simulink model "LaneFollowingNMPCWarda"  (R2021b)
settings: Solver=VariableStepAuto  StartTime=0.0  StopTime=Duration  FixedStep=0.1  RelTol=1e-3
PreLoadFcn:
  | LaneFollowingUsingNMPCData
undefined symbols (not defined in the file or in its folder): Cf, Cr, Iz, lf, lr, m, rho, tau, Ts, v0, v_set
libraries: fuzblock x6, mpclib x1, sharedTrackingLibrary x1
settings Model: NumberOfSteps=3  Creator=The MathWorks, Inc.  LastModifiedBy=Lenovo
settings SolverCC: AlgebraicLoopSolver=TrustRegion
settings DataIOCC: ExternalInput=[t curvature]  ReturnWorkspaceOutputs=off
settings DebuggingCC: PregeneratedLibrarySubsystemCodeDiagnostic=none  SFMachineParentedDataDiag=warning  ArithmeticOperatorsInVariantConditions=warning
settings SFSimCC: SimUseLocalCustomCode=off  CustomCodeUndefinedFunction=UseInterfaceOnly
settings RTWCC: RTWUseLocalCustomCode=off
settings CodeAppCC: StateflowObjectComments=on
settings SimscapeCC: SimscapeNormalizeSystem=off

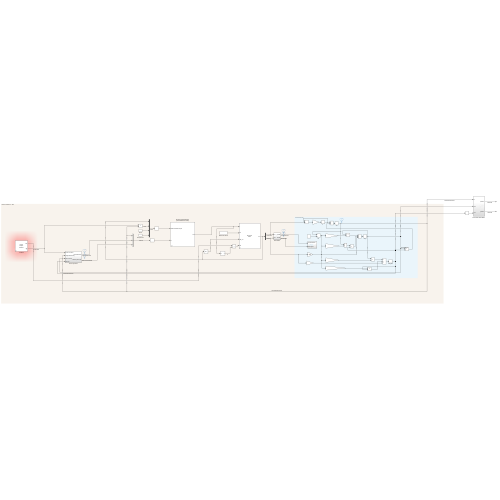
[thumbnail: Simulink's stored preview of the top-level diagram]
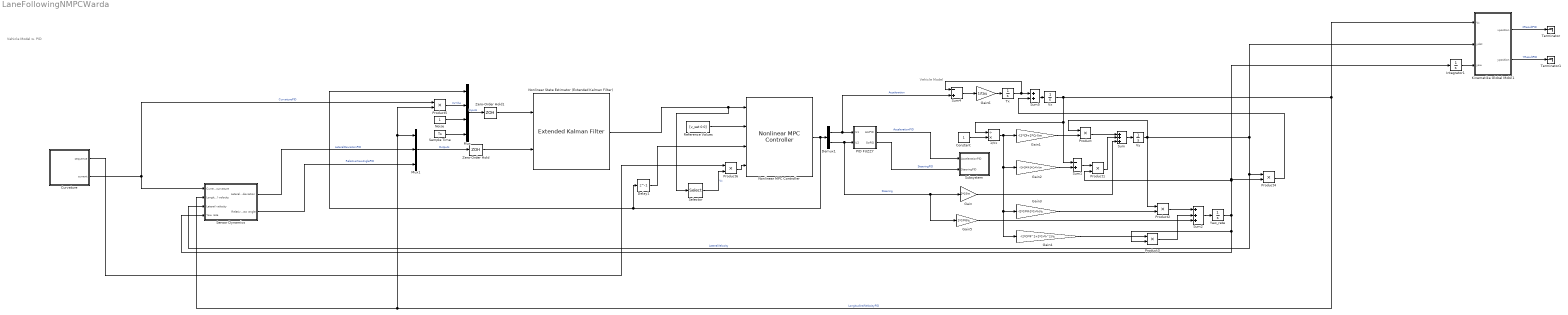
== system LaneFollowingNMPCWarda ==
  note: Vehicle Model w. PID
  note: Vehicle Model
  1/Vx : Product  Inputs=/*
  Constant : Constant
  Curvature : Subsystem  mask{signal=rho, ts=Ts, steps=10}
      mask prompts: signal "Signal name"; ts "Sampling time"; steps "Number of previewing steps"
      mask init:
      | ts = evalin('base',get_param(gcbh,'ts'));
      | signal = evalin('base',get_param(gcbh,'signal'));
      | steps = evalin('base',get_param(gcbh,'steps'));
      | data = mpc_previewer_maskinit(signal,ts);
      mask Display:
      | fprintf('Future\nsample\nextractor');
      | port_label('output', 1, 'seq')
      | port_label('output', 2, '@t')
  Delay1 : Delay  DelayLength=1  InitialCondition=[0.2 0.3]
  Demux1 : Demux  Outputs=2
  Gain : Gain  Gain=2*Cf/m
  Gain1 : Gain  Gain=-(2*Cf+2*Cr)/m
  Gain2 : Gain  Gain=-(2*Cf*lf-2*Cr*lr)/m
  Gain3 : Gain  Gain=-(2*Cf*lf-2*Cr*lr)/Iz
  Gain4 : Gain  Gain=-(2*Cf*lf^2+2*Cr*lr^2)/Iz
  Gain5 : Gain  Gain=2*Cf*lf/Iz
  Gain6 : Gain  Gain=1/tau
  Integrator1 : Integrator
  Kinematika Global Mobil1 : Subsystem
  Mux : Mux
  Mux1 : Mux  Inputs=3
  Noise : Constant
  Nonlinear MPC Controller : mpclib/Nonlinear MPC Controller  SCDEnableBlockLinearizationSpecification=on  nlmpcobj=nlobj  UseObjectTs=on  TsControl=Ts  UseMEX=off  md_enabled=on  mvtarget_enabled=off  param_enabled=off  cost_enabled=off  mvseq_enabled=off  stateseq_enabled=off  ovseq_enabled=off  slack_enabled=off  status_enabled=off  ov_min=off  ov_max=off  mv_min=off  mv_max=off  mvrate_min=off  mvrate_max=off  state_min=off  state_max=off  ov_weight=off  mv_weight=off  mvrate_weight=off  ecr_weight=off  nlp_initialize=off
  Nonlinear State Estimator (Extended Kalman Filter) : sharedTrackingLibrary/Extended Kalman Filter  StateTransitionFcn=LaneFollowingEKFStateFcn  HasStateTransitionJacobianFcn=off  HasAdditiveProcessNoise=Additive  ProcessNoise=1e-4*eye(7)  HasTimeVaryingProcessNoise=off  HasStateTransitionFcnExtraArgument=1  InitialState=[0 0 v0 0 0 0 0]'  InitialStateCovariance=1e-4*eye(7)  MeasurementFcn1=LaneFollowingEKFMeasFcn  HasMeasurementJacobianFcn1=off  HasMeasurementEnablePort1=off  HasAdditiveMeasurementNoise1=Additive  MeasurementNoise1=1e-4*eye(3)  HasTimeVaryingMeasurementNoise1=off  HasMeasurementFcnExtraArgument1=0  MeasurementFcn2=myMeasurementFcn  HasMeasurementJacobianFcn2=off  HasMeasurementEnablePort2=off  HasAdditiveMeasurementNoise2=Additive  MeasurementNoise2=1  HasTimeVaryingMeasurementNoise2=off  HasMeasurementFcnExtraArgument2=0  MeasurementFcn3=myMeasurementFcn  HasMeasurementJacobianFcn3=off  HasMeasurementEnablePort3=off  HasAdditiveMeasurementNoise3=Additive  MeasurementNoise3=1  HasTimeVaryingMeasurementNoise3=off  HasMeasurementFcnExtraArgument3=0  MeasurementFcn4=myMeasurementFcn  HasMeasurementJacobianFcn4=off  HasMeasurementEnablePort4=off  HasAdditiveMeasurementNoise4=Additive  MeasurementNoise4=1  HasTimeVaryingMeasurementNoise4=off  HasMeasurementFcnExtraArgument4=0  MeasurementFcn5=myMeasurementFcn  HasMeasurementJacobianFcn5=off  HasMeasurementEnablePort5=off  HasAdditiveMeasurementNoise5=Additive  MeasurementNoise5=1  HasTimeVaryingMeasurementNoise5=off  HasMeasurementFcnExtraArgument5=0  EnableMultirate=off  StateTransitionFcnSampleTime=1  MeasurementFcn1SampleTime=1  MeasurementFcn2SampleTime=1  MeasurementFcn3SampleTime=1  MeasurementFcn4SampleTime=1  MeasurementFcn5SampleTime=1  UseCurrentEstimator=on  OutputStateCovariance=off  DataType=double  SampleTime=Ts  NumberOfMeasurements=1
      settings: SourceProductBaseCode=AE,PW,CT,DR,TF,ID,LP,NV,AR,RO,RR,UV,VE
  PID FUZZY : Subsystem
  Product{,1..6} (7 alike) : Product
  Reference Values : Constant  Value=[v_set 0 0]  VectorParams1D=off
  Sample Time : Constant  Value=Ts
  Selector : Selector  InputPortWidth=7  IndexOptions=Index vector (dialog)  Indices=[3]  OutputSizes=1
  Sensor Dynamics : Subsystem
  Subsystem : Subsystem
  Sum : Sum  Inputs=+++
  Sum1 : Sum  Inputs=-+
  Sum2 : Sum  Inputs=+++
  Sum4 : Sum  Inputs=-+
  Sum5 : Sum
  Terminator : Terminator
  Terminator1 : Terminator
  Tx : Integrator
  Vx : Integrator  InitialCondition=v0
  Vy : Integrator
  "Yaw_rate " : Integrator
  Zero-Order Hold : ZeroOrderHold  SampleTime=Ts
  Zero-Order Hold1 : ZeroOrderHold  SampleTime=Ts
  wires:
  Curvature/2(current) -> Product5/1, Sensor Dynamics/1(Current curvature)  "CurvaturePID"
  "Yaw_rate "/1 -> Sensor Dynamics/4(Yaw rate), Product3/2, Integrator1/1, Product4/2, Product1/2
  Sensor Dynamics/1(Lateral deviation) -> Mux1/2  "LateralDeviationPID"
  Sensor Dynamics/2(Relative yaw angle) -> Mux1/3  "RelativeYawAnglePID"
  Sum5/1 -> Vx/1
  Product1/1 -> Sum/2
  Gain1/1 -> Product/2
  Gain6/1 -> Tx/1
  Product/1 -> Sum/1
  Tx/1 -> Sum5/1, Sum4/1
  Sum/1 -> Vy/1
  Product2/1 -> Sum2/1
  1/Vx/1 -> Gain4/1, Gain3/1, Gain2/1, Gain1/1
  Gain/1 -> Sum/3
  Sum1/1 -> Product1/1
  Gain5/1 -> Sum2/3
  Product4/1 -> Sum5/2
  Constant/1 -> 1/Vx/2
  Sum4/1 -> Gain6/1
  Gain4/1 -> Product3/1
  Product3/1 -> Sum2/2
  Gain3/1 -> Product2/2
  Sum2/1 -> "Yaw_rate "/1
  Gain2/1 -> Sum1/2
  Zero-Order Hold1/1 -> Nonlinear State Estimator (Extended Kalman Filter)/1
  Product5/1 -> Mux/2  "Vx*rho"
  Zero-Order Hold/1 -> Nonlinear State Estimator (Extended Kalman Filter)/2
  Mux/1 -> Zero-Order Hold1/1  "Inputs"
  Nonlinear MPC Controller/1 -> Mux/1, Delay1/1, Demux1/1
  Sample Time/1 -> Mux/4
  Mux1/1 -> Zero-Order Hold/1  "Outputs"
  Noise/1 -> Mux/3
  Curvature/1(sequence) -> Product6/1
  Nonlinear State Estimator (Extended Kalman Filter)/1 -> Selector/1, Nonlinear MPC Controller/1
  Selector/1 -> Product6/2  "Vx"
  Product6/1 -> Nonlinear MPC Controller/4
  Reference Values/1 -> Nonlinear MPC Controller/2
  Delay1/1 -> Nonlinear MPC Controller/3
  Demux1/1 -> Sum4/2, PID FUZZY/1(U1)  "Acceleration"
  Demux1/2 -> Gain5/1, Gain/1, PID FUZZY/2(U2)  "Steering"
  Kinematika Global Mobil1/2(yposition) -> Terminator1/1  "YResultPID"
  Kinematika Global Mobil1/1(xposition) -> Terminator/1  "XResultPID"
  Integrator1/1 -> Kinematika Global Mobil1/3(yaw)
  Vx/1 -> Mux1/1, Product5/2, Sensor Dynamics/2(Longitudinal velocity), Kinematika Global Mobil1/1(Vx), 1/Vx/1, Sum1/1  "LongitudinalVelocityPID"
  Vy/1 -> Product/1, Sensor Dynamics/3(Lateral velocity), Product4/1, Kinematika Global Mobil1/2(ydot), Product2/1  "LateralVelocity"
  PID FUZZY/1(AccPID) -> Subsystem/1(AccelerationPID)  "AccelerationPID"
  PID FUZZY/2(StrPID) -> Subsystem/2(SteeringPID)  "SteeringPID"

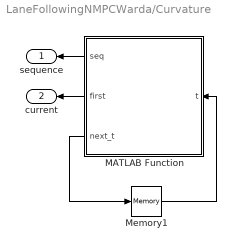
== system LaneFollowingNMPCWarda/Curvature ==
  MATLAB Function : MATLAB Function  TreatAsAtomicUnit=on
  Memory1 : Memory  InheritSampleTime=on  LinearizeAsDelay=on
  sequence : Outport  VectorParamsAs1DForOutWhenUnconnected=off
  current : Outport  Port=2  VectorParamsAs1DForOutWhenUnconnected=off
  wires:
  MATLAB Function/1(seq) -> sequence/1
  MATLAB Function/2(first) -> current/1
  Memory1/1 -> MATLAB Function/1(t)
  MATLAB Function/3(next_t) -> Memory1/1

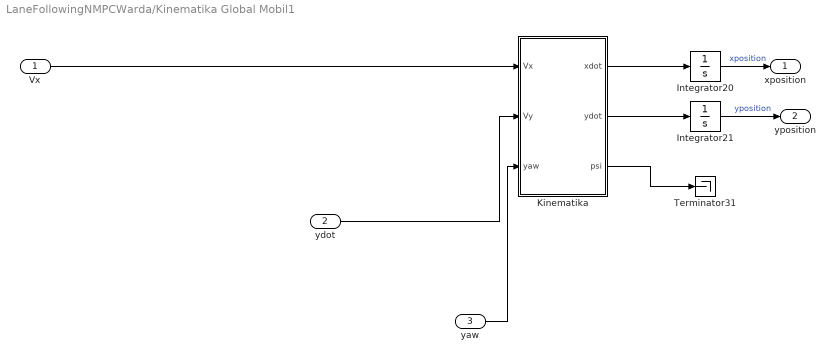
== system LaneFollowingNMPCWarda/Kinematika Global Mobil1 ==
  Vx : Inport
  ydot : Inport  Port=2
  yaw : Inport  Port=3
  Integrator20 : Integrator  InitialCondition=-77.3002666917596
  Integrator21 : Integrator  InitialCondition=1.57171568074885
  Kinematika : MATLAB Function  TreatAsAtomicUnit=on
  Terminator31 : Terminator
  xposition : Outport
  yposition : Outport  Port=2
  wires:
  Kinematika/1(xdot) -> Integrator20/1
  Integrator20/1 -> xposition/1  "xposition"
  Kinematika/2(ydot) -> Integrator21/1
  Integrator21/1 -> yposition/1  "yposition"
  Vx/1 -> Kinematika/1(Vx)
  ydot/1 -> Kinematika/2(Vy)
  Kinematika/3(psi) -> Terminator31/1
  yaw/1 -> Kinematika/3(yaw)

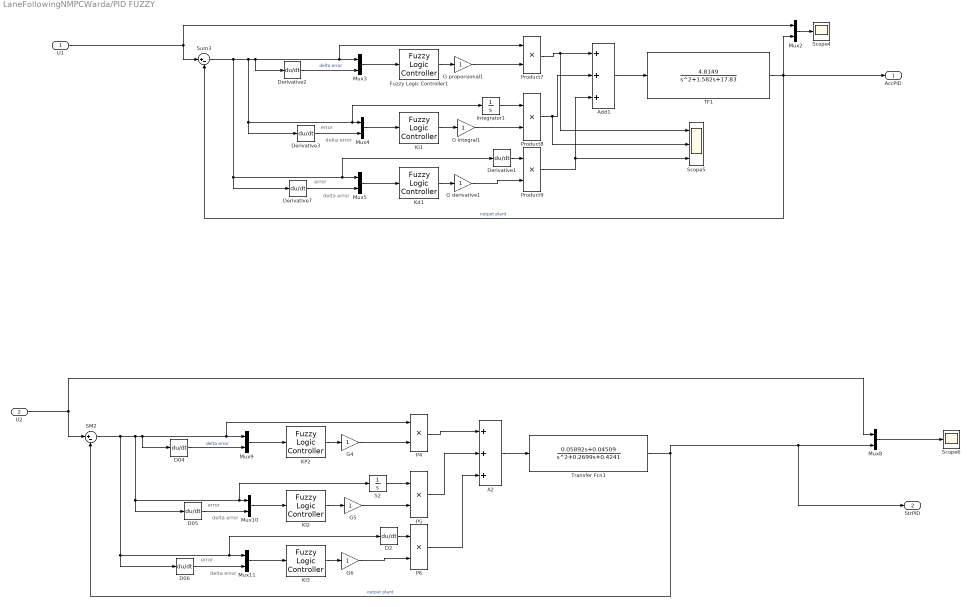
== system LaneFollowingNMPCWarda/PID FUZZY ==
  note: error
  note: delta error
  note: error
  note: delta error
  note: delta error
  note: error
  note: error
  note: delta error
  U1 : Inport
  U2 : Inport  Port=2
  A2 : Sum  Inputs=+++
  Add1 : Sum  Inputs=+++
  D04 : Derivative
  D05 : Derivative
  D06 : Derivative
  D2 : Derivative
  Derivative{1..3,7} (4 alike) : Derivative
  Fuzzy Logic Controller1 : fuzblock/Fuzzy Logic  Controller  FIS='Kp_pos2.fis'  OutputSampleNumber=101  DataType=double  FuzzifiedInputs=off  RuleFiringStrengths=off  RuleOutputs=off  AggregatedOutputs=off  SimulateUsing=Interpreted execution  OutOfRangeInputValueMessage=none  NoRuleFiredMessage=none  EmptyOutputFuzzySetMessage=none
  G derivative1 : Gain
  G integral1 : Gain
  G proporsional1 : Gain
  G4 : Gain
  G5 : Gain
  G6 : Gain
  Integrator1 : Integrator
  KI2 : fuzblock/Fuzzy Logic  Controller  FIS='Ki_pos3.fis'  OutputSampleNumber=101  DataType=double  FuzzifiedInputs=off  RuleFiringStrengths=off  RuleOutputs=off  AggregatedOutputs=off  SimulateUsing=Interpreted execution  OutOfRangeInputValueMessage=none  NoRuleFiredMessage=none  EmptyOutputFuzzySetMessage=none
  KI3 : fuzblock/Fuzzy Logic  Controller  FIS='Kd_pos.fis'  OutputSampleNumber=101  DataType=double  FuzzifiedInputs=off  RuleFiringStrengths=off  RuleOutputs=off  AggregatedOutputs=off  SimulateUsing=Interpreted execution  OutOfRangeInputValueMessage=none  NoRuleFiredMessage=none  EmptyOutputFuzzySetMessage=none
  KP2 : fuzblock/Fuzzy Logic  Controller  FIS='Kp_pos.fis'  OutputSampleNumber=101  DataType=double  FuzzifiedInputs=off  RuleFiringStrengths=off  RuleOutputs=off  AggregatedOutputs=off  SimulateUsing=Interpreted execution  OutOfRangeInputValueMessage=none  NoRuleFiredMessage=none  EmptyOutputFuzzySetMessage=none
  Kd1 : fuzblock/Fuzzy Logic  Controller  FIS='Kd_pos.fis'  OutputSampleNumber=101  DataType=double  FuzzifiedInputs=off  RuleFiringStrengths=off  RuleOutputs=off  AggregatedOutputs=off  SimulateUsing=Interpreted execution  OutOfRangeInputValueMessage=none  NoRuleFiredMessage=none  EmptyOutputFuzzySetMessage=none
  Ki1 : fuzblock/Fuzzy Logic  Controller  FIS='Ki_pos3.fis'  OutputSampleNumber=101  DataType=double  FuzzifiedInputs=off  RuleFiringStrengths=off  RuleOutputs=off  AggregatedOutputs=off  SimulateUsing=Interpreted execution  OutOfRangeInputValueMessage=none  NoRuleFiredMessage=none  EmptyOutputFuzzySetMessage=none
  Mux{2..5,8..11} (8 alike) : Mux  Inputs=2
  P4 : Product
  P5 : Product
  P6 : Product
  Product7 : Product
  Product8 : Product
  Product9 : Product
  S2 : Integrator
  SM2 : Sum  Inputs=|+-
  Scope4 : Scope
  Scope5 : Scope  NumInputPorts=3
  Scope6 : Scope
  Sum3 : Sum  Inputs=|+-
  TF1 : TransferFcn  Numerator=[4.8149]  Denominator=[1 1.582 17.83]
  Transfer Fcn1 : TransferFcn  Numerator=[0.05892 0.04509]  Denominator=[1 0.2699 0.4241]
  AccPID : Outport
  StrPID : Outport  Port=2
  wires:
  Derivative1/1 -> Product9/1
  Fuzzy Logic Controller1/1 -> G proporsional1/1
  U2/1 -> SM2/1, Mux8/1
  TF1/1 -> Mux2/2, AccPID/1, Sum3/2  "output plant"
  Product8/1 -> Scope5/2, Add1/2
  Sum3/1 -> Derivative7/1, Derivative1/1, Mux5/1, Derivative3/1, Integrator1/1, Mux4/1, Derivative2/1, Product7/1, Mux3/1
  SM2/1 -> D06/1, D2/1, Mux11/1, D05/1, S2/1, Mux10/1, D04/1, P4/1, Mux9/1
  A2/1 -> Transfer Fcn1/1
  Ki1/1 -> G integral1/1
  D04/1 -> Mux9/2  "delta error"
  Mux8/1 -> Scope6/1
  G proporsional1/1 -> Product7/2
  Product9/1 -> Scope5/3, Add1/3
  Integrator1/1 -> Product8/1
  Mux9/1 -> KP2/1
  P6/1 -> A2/3
  Mux11/1 -> KI3/1
  KP2/1 -> G4/1
  Product7/1 -> Scope5/1, Add1/1
  Kd1/1 -> G derivative1/1
  Mux10/1 -> KI2/1
  Derivative2/1 -> Mux3/2  "delta error"
  G integral1/1 -> Product8/2
  G derivative1/1 -> Product9/2
  Mux3/1 -> Fuzzy Logic Controller1/1
  Mux5/1 -> Kd1/1
  D05/1 -> Mux10/2
  Add1/1 -> TF1/1
  U1/1 -> Sum3/1, Mux2/1
  Mux2/1 -> Scope4/1
  D06/1 -> Mux11/2
  G6/1 -> P6/2
  Mux4/1 -> Ki1/1
  G4/1 -> P4/2
  P4/1 -> A2/1
  Transfer Fcn1/1 -> SM2/2, StrPID/1, Mux8/2  "output plant"
  KI3/1 -> G6/1
  D2/1 -> P6/1
  G5/1 -> P5/2
  KI2/1 -> G5/1
  Derivative7/1 -> Mux5/2
  Derivative3/1 -> Mux4/2
  P5/1 -> A2/2
  S2/1 -> P5/1

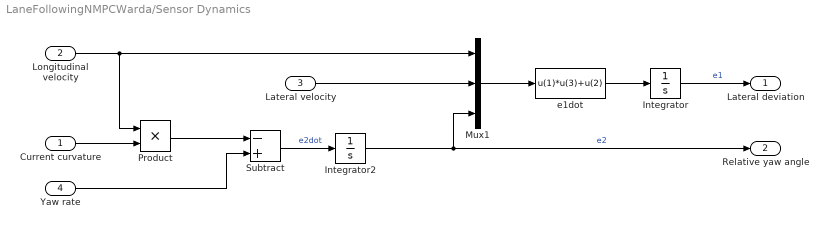
== system LaneFollowingNMPCWarda/Sensor Dynamics ==
  Current curvature : Inport
  Longitudinal velocity : Inport  Port=2
  Lateral velocity : Inport  Port=3
  Yaw rate : Inport  Port=4
  Integrator : Integrator
  Integrator2 : Integrator
  Mux1 : Mux  Inputs=[1 1 1]
  Product : Product
  Subtract : Sum  Inputs=-+
  e1dot : Fcn  Expr=u(1)*u(3)+u(2)
  Lateral deviation : Outport  VectorParamsAs1DForOutWhenUnconnected=off
  Relative yaw angle : Outport  Port=2  VectorParamsAs1DForOutWhenUnconnected=off
  wires:
  Current curvature/1 -> Product/2
  Mux1/1 -> e1dot/1
  e1dot/1 -> Integrator/1
  Longitudinal velocity/1 -> Product/1, Mux1/1
  Lateral velocity/1 -> Mux1/2
  Integrator/1 -> Lateral deviation/1  "e1"
  Product/1 -> Subtract/1
  Yaw rate/1 -> Subtract/2
  Subtract/1 -> Integrator2/1  "e2dot"
  Integrator2/1 -> Mux1/3, Relative yaw angle/1  "e2"

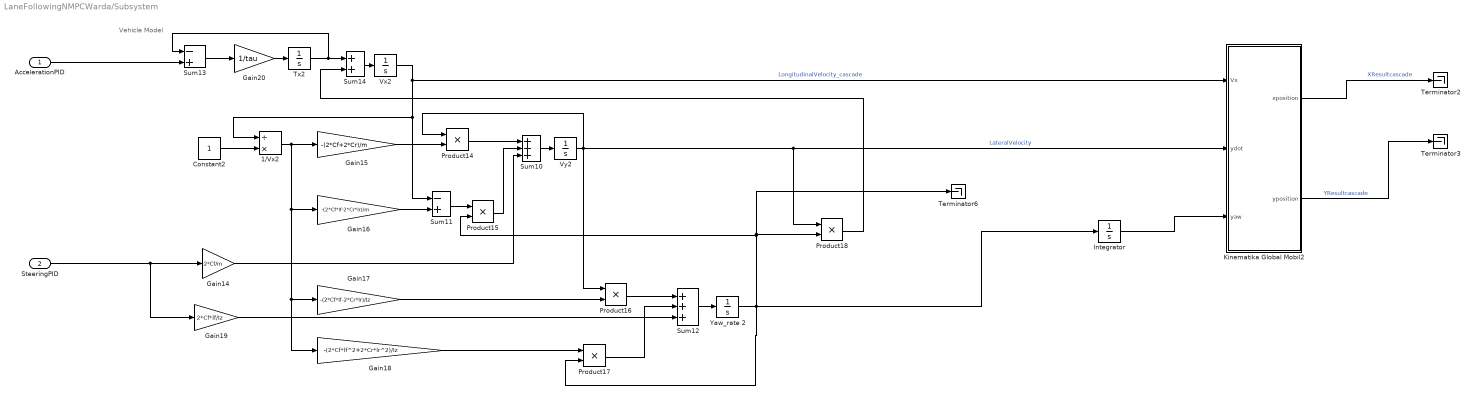
== system LaneFollowingNMPCWarda/Subsystem ==
  note: Vehicle Model
  AccelerationPID : Inport
  SteeringPID : Inport  Port=2
  1/Vx2 : Product  Inputs=/*
  Constant2 : Constant
  Gain14 : Gain  Gain=2*Cf/m
  Gain15 : Gain  Gain=-(2*Cf+2*Cr)/m
  Gain16 : Gain  Gain=-(2*Cf*lf-2*Cr*lr)/m
  Gain17 : Gain  Gain=-(2*Cf*lf-2*Cr*lr)/Iz
  Gain18 : Gain  Gain=-(2*Cf*lf^2+2*Cr*lr^2)/Iz
  Gain19 : Gain  Gain=2*Cf*lf/Iz
  Gain20 : Gain  Gain=1/tau
  Integrator : Integrator
  Kinematika Global Mobil2 : Subsystem
  Product{14..18} (5 alike) : Product
  Sum10 : Sum  Inputs=+++
  Sum11 : Sum  Inputs=-+
  Sum12 : Sum  Inputs=+++
  Sum13 : Sum  Inputs=-+
  Sum14 : Sum
  Terminator2 : Terminator
  Terminator3 : Terminator
  Terminator6 : Terminator
  Tx2 : Integrator
  Vx2 : Integrator  InitialCondition=v0
  Vy2 : Integrator
  Yaw_rate 2 : Integrator
  wires:
  Sum10/1 -> Vy2/1
  Gain14/1 -> Sum10/3
  Sum13/1 -> Gain20/1
  Tx2/1 -> Sum14/1, Sum13/1
  Yaw_rate 2/1 -> Integrator/1, Product17/2, Terminator6/1, Product18/2, Product15/2
  AccelerationPID/1 -> Sum13/2
  Sum14/1 -> Vx2/1
  Vy2/1 -> Product14/1, Kinematika Global Mobil2/2(ydot), Product18/1, Product16/1  "LateralVelocity"
  Product18/1 -> Sum14/2
  Gain15/1 -> Product14/2
  Gain20/1 -> Tx2/1
  Product14/1 -> Sum10/1
  Product15/1 -> Sum10/2
  Product17/1 -> Sum12/2
  Sum12/1 -> Yaw_rate 2/1
  Gain19/1 -> Sum12/3
  Product16/1 -> Sum12/1
  1/Vx2/1 -> Gain18/1, Gain17/1, Gain16/1, Gain15/1
  Gain16/1 -> Sum11/2
  Gain18/1 -> Product17/1
  Constant2/1 -> 1/Vx2/2
  Sum11/1 -> Product15/1
  Gain17/1 -> Product16/2
  SteeringPID/1 -> Gain19/1, Gain14/1
  Vx2/1 -> Kinematika Global Mobil2/1(Vx), 1/Vx2/1, Sum11/1  "LongitudinalVelocity_cascade"
  Kinematika Global Mobil2/2(yposition) -> Terminator3/1  "YResultcascade"
  Kinematika Global Mobil2/1(xposition) -> Terminator2/1  "XResultcascade"
  Integrator/1 -> Kinematika Global Mobil2/3(yaw)

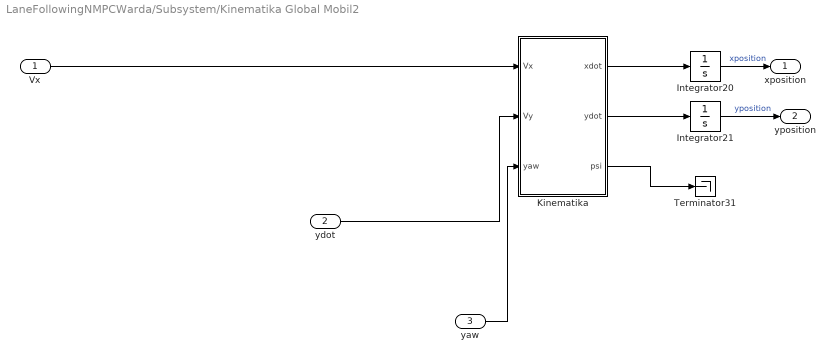
== system LaneFollowingNMPCWarda/Subsystem/Kinematika Global Mobil2 ==
  Vx : Inport
  ydot : Inport  Port=2
  yaw : Inport  Port=3
  Integrator20 : Integrator  InitialCondition=-77.3002666917596
  Integrator21 : Integrator  InitialCondition=1.57171568074885
  Kinematika : MATLAB Function  TreatAsAtomicUnit=on
  Terminator31 : Terminator
  xposition : Outport
  yposition : Outport  Port=2
  wires:
  Kinematika/1(xdot) -> Integrator20/1
  Integrator20/1 -> xposition/1  "xposition"
  Kinematika/2(ydot) -> Integrator21/1
  Integrator21/1 -> yposition/1  "yposition"
  Vx/1 -> Kinematika/1(Vx)
  ydot/1 -> Kinematika/2(Vy)
  Kinematika/3(psi) -> Terminator31/1
  yaw/1 -> Kinematika/3(yaw)

== matlab function LaneFollowingNMPCWarda/Curvature/MATLAB Function ==
  settings: updateMethod=DISCRETE  sampleTime=ts
  data: data parameter; seq output; steps parameter; t input; first output; next_t output
function [seq,first,next_t] = fcn(data,steps,t)
%#codegen
[seq,first,next_t] = mpcblock_preview('md',data,steps,t);

== matlab function LaneFollowingNMPCWarda/Kinematika Global Mobil1/Kinematika ==
  data: Vx input; Vy input; yaw input; xdot output; ydot output; psi output
function [xdot,ydot,psi] = fcn(Vx,Vy,yaw)
a = yaw;
xdot = Vx*cos(a)-Vy*sin(a);
ydot = Vx*sin(a)+Vy*cos(a);
psi = a;

== matlab function LaneFollowingNMPCWarda/Subsystem/Kinematika Global Mobil2/Kinematika ==
  data: Vx input; Vy input; yaw input; xdot output; ydot output; psi output
function [xdot,ydot,psi] = fcn(Vx,Vy,yaw)
a = yaw;
xdot = Vx*cos(a)-Vy*sin(a);
ydot = Vx*sin(a)+Vy*cos(a);
psi = a;
